simulink library "SHUTDOWN"  (Simulink 8.6)
settings: Solver=VariableStepAuto  StartTime=0.0  StopTime=10.0  RelTol=1e-3
libraries: cdsEpicsOut x4, cdsModelRate x1, cdsFunctionCall x1, cdsEpicsIn x1
settings Model: Creator=controls  LastModifiedBy=controls

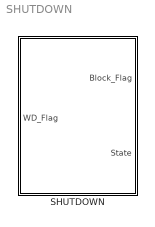
== system SHUTDOWN ==
  SHUTDOWN : Subsystem

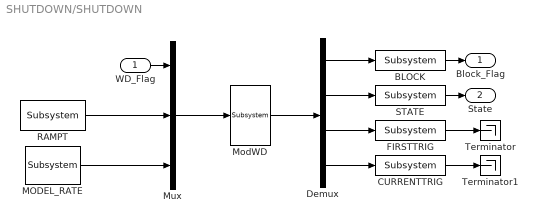
== system SHUTDOWN/SHUTDOWN ==
  WD_Flag : Inport
  BLOCK : cdsEpicsOut/Subsystem  Tag=cdsEpicsOutput  Description=|
      | Purpose:                                          
      | Output a FE signal to an EPICS channel.           
      |                                                   
      | Operation:                                        
      | Takes input value and passes it to EPICS record.  
      |                                                   
      | Usage:                                            
      | Name the part with the desired EPICS rrecord name.
      settings: AttributesFormatString=%<Tag>
  CURRENTTRIG : cdsEpicsOut/Subsystem  Tag=cdsEpicsOutput  Description=|
      | Purpose:                                          
      | Output a FE signal to an EPICS channel.           
      |                                                   
      | Operation:                                        
      | Takes input value and passes it to EPICS record.  
      |                                                   
      | Usage:                                            
      | Name the part with the desired EPICS rrecord name.
      settings: AttributesFormatString=%<Tag>
  Demux : Demux
  FIRSTTRIG : cdsEpicsOut/Subsystem  Tag=cdsEpicsOutput  Description=|
      | Purpose:                                          
      | Output a FE signal to an EPICS channel.           
      |                                                   
      | Operation:                                        
      | Takes input value and passes it to EPICS record.  
      |                                                   
      | Usage:                                            
      | Name the part with the desired EPICS rrecord name.
      settings: AttributesFormatString=%<Tag>
  MODEL_RATE : cdsModelRate/Subsystem  Tag=cdsModelRate
      settings: AttributesFormatString=%<Tag>
  ModWD : cdsFunctionCall/Subsystem  Tag=cdsFunctionCall  Description=inline ModerateWD /opt/rtcds/userapps/release/vis/common/src/ModerateWD.c
      settings: AttributesFormatString=%<Tag>
  Mux : Mux  Inputs=3
  RAMPT : cdsEpicsIn/Subsystem  Tag=cdsEpicsIn  Description=|
      | Purpose:                                                                              
      | Create an EPICS input channel connection to the FE realtime controls.                 
      |                                                                                       
      | Operation:                                                                            
      | Outputs value from an EPICS ai record. Value is floating point with a precision of 3..
      |                                                                                       
      | Usage:                                                                                
      | Name the part with the desired EPICS channel name.
      settings: AttributesFormatString=%<Tag>
  STATE : cdsEpicsOut/Subsystem  Tag=cdsEpicsOutput  Description=|
      | Purpose:                                          
      | Output a FE signal to an EPICS channel.           
      |                                                   
      | Operation:                                        
      | Takes input value and passes it to EPICS record.  
      |                                                   
      | Usage:                                            
      | Name the part with the desired EPICS rrecord name.
      settings: AttributesFormatString=%<Tag>
  Terminator : Terminator
  Terminator1 : Terminator
  Block_Flag : Outport
  State : Outport  Port=2
  wires:
  RAMPT/1 -> Mux/2
  FIRSTTRIG/1 -> Terminator/1
  Demux/1 -> BLOCK/1
  Demux/2 -> STATE/1
  Demux/4 -> CURRENTTRIG/1
  Demux/3 -> FIRSTTRIG/1
  STATE/1 -> State/1
  CURRENTTRIG/1 -> Terminator1/1
  WD_Flag/1 -> Mux/1
  BLOCK/1 -> Block_Flag/1
  MODEL_RATE/1 -> Mux/3
  ModWD/1 -> Demux/1
  Mux/1 -> ModWD/1
